simulink model "simul_same"  (R2020b)
settings: Solver=VariableStepAuto  StartTime=0.0  StopTime=10.0  RelTol=1e-3
libraries: cstblocks x4
settings Model: Creator=kisel  LastModifiedBy=kisel

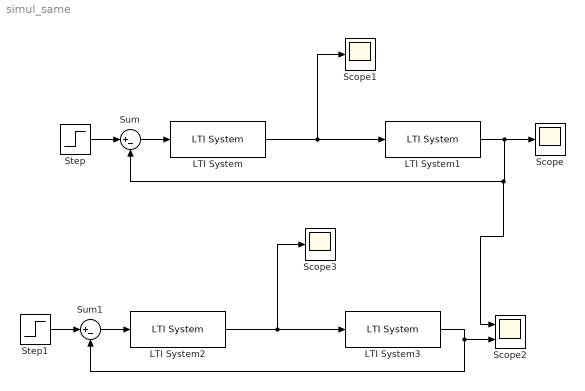
== system simul_same ==
  LTI System : cstblocks/LTI System  sys=Dc  IC=[]
  LTI System1 : cstblocks/LTI System  sys=D  IC=[]
  LTI System2 : cstblocks/LTI System  sys=Dc  IC=[]
  LTI System3 : cstblocks/LTI System  sys=W  IC=[]
  Scope : Scope
  Scope1 : Scope
  Scope2 : Scope  NumInputPorts=2
  Scope3 : Scope
  Step : Step  Time=0  SampleTime=0
  Step1 : Step  Time=0  SampleTime=0
  Sum : Sum  Inputs=|+-
  Sum1 : Sum  Inputs=|+-
  wires:
  LTI System/1 -> Scope1/1, LTI System1/1
  Sum/1 -> LTI System/1
  LTI System1/1 -> Scope/1, Scope2/1, Sum/2
  Step/1 -> Sum/1
  LTI System3/1 -> Scope2/2, Sum1/2
  Sum1/1 -> LTI System2/1
  LTI System2/1 -> Scope3/1, LTI System3/1
  Step1/1 -> Sum1/1
